simulink model "simulation"  (R2018b)
settings: Solver=VariableStepAuto  StartTime=0.0  StopTime=100  RelTol=1e-3
values from neighbouring files (symbols this model uses):
  x_IC = [0 ... (first row only)    [script_sim.m]
settings Model: Creator=claud  LastModifiedBy=claud

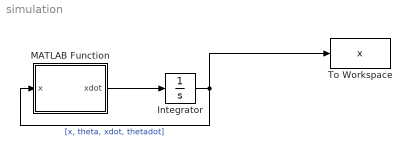
== system simulation ==
  Integrator : Integrator  InitialCondition=x_IC
  MATLAB Function : MATLAB Function  TreatAsAtomicUnit=on
  To Workspace : ToWorkspace  VariableName=x  SampleTime=-1
  wires:
  MATLAB Function/1(xdot) -> Integrator/1
  Integrator/1 -> MATLAB Function/1(x), To Workspace/1  "[x, theta, xdot, thetadot]"

== matlab function simulation/MATLAB Function ==
  data: xdot output; x input
function xdot  = fcn (x)

mw = .222;     % Mass of wheel (kg)
mb = 1.179;    % Mass of body (kg)
rw = .005;     % Radius of wheel (m)
rb = .349;     % Distance from center of wheel to c.g. of body (m)
Iwyy = 1*10^-5;
Ibyy = 1*10^-5;
Tm = 0.1;
g = 9.81; 

mx = mb + (2*mw) + (2*(Iwyy / (rw*rw)));
I_theta = (mb*rb*rb) + Ibyy;

c = cos(x(1));
s = sin(x(1));

A = [[1, 0, 0, 0];
    [0,1,0,0];
    [0,0, mx, mb*rb*c]; 
    [0,0,mb*rb*c, I_theta]];

b = [x(3);
     x(4); 
    (2* Tm) / (rw + (mb*rb*s*x(4)^2)); 
     2*Tm + (mb * rb * s * g)];
    

xdot = A \ b;
